simulink model "radia_streamfunction_optimization"  (R2026a)
settings: Solver=FixedStepDiscrete  StopTime=1  FixedStep=1
model workspace (MAT data in the model file):
  radia_streamfunction_adjoint_runner = radia.topopt.AdjointRunner
  radia_streamfunction_adjoint_runner.InitialDesign = [0.7; 0.7]
  radia_streamfunction_adjoint_runner.EvaluateFcn : function handle (value not decoded)
  radia_streamfunction_adjoint_runner.Options.LowerBounds = [0; 0]
  radia_streamfunction_adjoint_runner.Options.UpperBounds = [1; 1]
  radia_streamfunction_adjoint_runner.Options.MaxIterations = 40
  radia_streamfunction_adjoint_runner.Options.MoveLimit = [0.2; 0.2]
  radia_streamfunction_adjoint_runner.Metadata.domain = "stream-function"
  radia_streamfunction_adjoint_runner.Metadata.parameterization = "stream-function-coefficients"
  radia_streamfunction_adjoint_runner.Metadata.gradient = "analytic-adjoint"
  radia_streamfunction_adjoint_runner.Metadata.response_count = 2
  radia_streamfunction_adjoint_runner.Metadata.design_count = 2
  radia_streamfunction_adjoint_runner.Metadata.current_constraint_count = 1
settings Model: Creator=administrator  LastModifiedBy=administrator

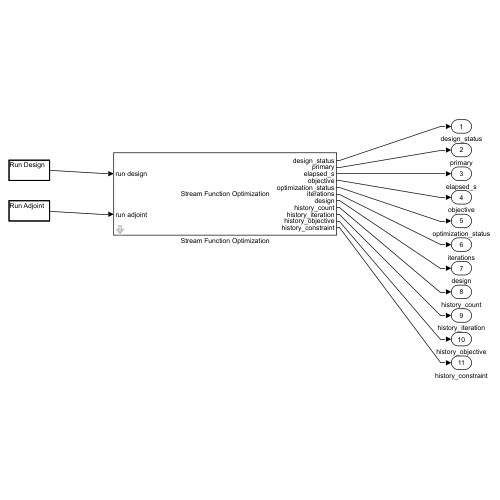
[thumbnail: Simulink's stored preview of the top-level diagram]
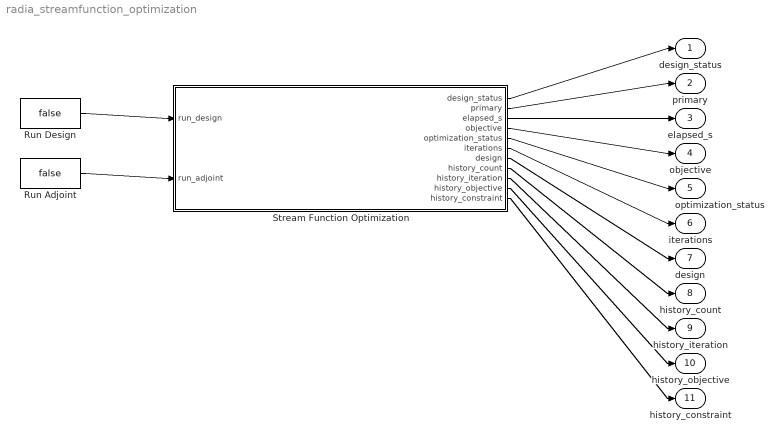
== system radia_streamfunction_optimization ==
  Run Adjoint : Constant  Value=false  OutDataTypeStr=boolean
  Run Design : Constant  Value=false  OutDataTypeStr=boolean
  Stream Function Optimization : Subsystem  mask{config_file='', run_root='C:\temp\radia_simulink', timeout_s=3600, python_executable='python', radia_streamfunction_adjoint_runner=radia_streamfunction_adjoint_runner, solver=mma, sample_time_s=1, history_capacity=64}
      mask prompts: config_file "Design configuration JSON"; run_root "Run artifact root"; timeout_s "Timeout (s)"; python_executable "Python executable"; radia_streamfunction_adjoint_runner "Stream-function adjoint runner"; solver "Optimizer"; sample_time_s "Sample time (s)"; history_capacity "History capacity"
      mask help: Stream-function design/Pareto batch plus analytic MMA/SQP coefficient optimization and Simulink-native history plots.
      mask init:
      | radia.simulink.configureStreamFunctionOptimizationSubsystem(gcb);
      mask TypeOptions solver: mma | sqp
      mask Display: disp('Stream Function Optimization');port_label('input',1,'run design');port_label('input',2,'run adjoint');port_label('output',1,'design_status');port_label('output',2,'primary');port_label('output',3,'elapsed_s');port_label('output',4,'objective');port_label('output',5,'optimization_status');port_label('output',6,'iterations');port_label('output',7,'design');port_label('output',8,'history_count');port_label('output',9,'history_iteration');port_label('output',10,'history_objective');port_label('output',11,'history_constraint');
  design_status : Outport
  primary : Outport  Port=2
  elapsed_s : Outport  Port=3
  objective : Outport  Port=4
  optimization_status : Outport  Port=5
  iterations : Outport  Port=6
  design : Outport  Port=7
  history_count : Outport  Port=8
  history_iteration : Outport  Port=9
  history_objective : Outport  Port=10
  history_constraint : Outport  Port=11
  wires:
  Run Design/1 -> Stream Function Optimization/1(run_design)
  Run Adjoint/1 -> Stream Function Optimization/2(run_adjoint)
  Stream Function Optimization/1(design_status) -> design_status/1
  Stream Function Optimization/2(primary) -> primary/1
  Stream Function Optimization/3(elapsed_s) -> elapsed_s/1
  Stream Function Optimization/4(objective) -> objective/1
  Stream Function Optimization/5(optimization_status) -> optimization_status/1
  Stream Function Optimization/6(iterations) -> iterations/1
  Stream Function Optimization/7(design) -> design/1
  Stream Function Optimization/8(history_count) -> history_count/1
  Stream Function Optimization/9(history_iteration) -> history_iteration/1
  Stream Function Optimization/10(history_objective) -> history_objective/1
  Stream Function Optimization/11(history_constraint) -> history_constraint/1

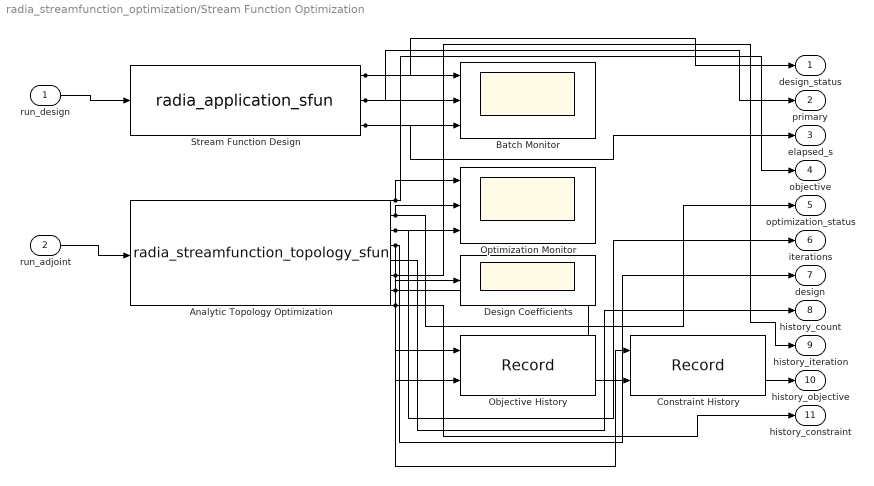
== system radia_streamfunction_optimization/Stream Function Optimization ==
  run_design : Inport  OutDataTypeStr=boolean
  run_adjoint : Inport  Port=2  OutDataTypeStr=boolean
  Analytic Topology Optimization : M-S-Function  FunctionName=radia_streamfunction_topology_sfun  Parameters=radia_streamfunction_adjoint_runner,1,64
  Batch Monitor : Scope  NumInputPorts=3
  Constraint History : Record  NumPorts=2.0  FileSettingsInternal="{\"entries\":[{\"content\":{\"excelSettings\":{\"content\":{},\"type\":\"Streamout.ExcelSettings\"},\"parquetSettings\":{\"content\":{},\"type\":\"Streamout.ParquetSettings\"}},\"type\":\"Streamout.FileSettingStorage\",\"uuid\":\"\"}],\"packageUris\":[\"http:\\/\\/schema.mathworks.com\\/mf0\\/streamout_blocks\\/R2020a\"],\"version\":\"1.0\"}"  FrameSettings=[0, 0]  Layout=[1 1]  SignalsInternal="{\"entries\":[{\"content\":{\"signals\":[{\"content\":{\"blockPath\":[],\"dimensions\":[1],\"domain\":\"\",\"lineColor\":\"#a2142f\",\"plots\":[ 1 ],\"port\":1,\"signalID\":1,\"signalName\":\"XY Graph:1\"},\"type\":\"RecordBlkView.Signal\",\"uuid\":\"\"},{\"content\":{\"blockPath\":[],\"dimensions\":[1],\"domain\":\"\",\"lineColor\":\"#139fff\",\"plots\":[ 1 ],\"port\":2,\"signalID\":2,\"signalName\":\"XY Graph:2\"},\"type\":\"RecordBlkView.Signal\",\"uuid\":\"\"}]},\"type\":\"RecordBlkView.InputSignals\",\"uuid\":\"\"}],\"packageUris\":[\"http:\\/\\/schema.mathworks.com\\/mf0\\/streamout_blocks\\/R2020a\"],\"version\":\"1.0\"}"  VisualizationBindings="{\"xyplotplugin\":{\"info\":[{\"series\":[{\"bindingParametersList\":[{\"parameter\":\"X-Axis\",\"signalID\":1,\"signalName\":\"XY Graph:1\"},{\"parameter\":\"Y-Axis\",\"signalID\":2,\"signalName\":\"XY Graph:2\"}],\"seriesID\":0}],\"subplotID\":1}]}}"  CompatibilityTag=XY
  Design Coefficients : Scope
  Objective History : Record  NumPorts=2.0  FileSettingsInternal="{\"entries\":[{\"content\":{\"excelSettings\":{\"content\":{},\"type\":\"Streamout.ExcelSettings\"},\"parquetSettings\":{\"content\":{},\"type\":\"Streamout.ParquetSettings\"}},\"type\":\"Streamout.FileSettingStorage\",\"uuid\":\"\"}],\"packageUris\":[\"http:\\/\\/schema.mathworks.com\\/mf0\\/streamout_blocks\\/R2020a\"],\"version\":\"1.0\"}"  FrameSettings=[0, 0]  Layout=[1 1]  SignalsInternal="{\"entries\":[{\"content\":{\"signals\":[{\"content\":{\"blockPath\":[],\"dimensions\":[1],\"domain\":\"\",\"lineColor\":\"#a2142f\",\"plots\":[ 1 ],\"port\":1,\"signalID\":1,\"signalName\":\"XY Graph:1\"},\"type\":\"RecordBlkView.Signal\",\"uuid\":\"\"},{\"content\":{\"blockPath\":[],\"dimensions\":[1],\"domain\":\"\",\"lineColor\":\"#139fff\",\"plots\":[ 1 ],\"port\":2,\"signalID\":2,\"signalName\":\"XY Graph:2\"},\"type\":\"RecordBlkView.Signal\",\"uuid\":\"\"}]},\"type\":\"RecordBlkView.InputSignals\",\"uuid\":\"\"}],\"packageUris\":[\"http:\\/\\/schema.mathworks.com\\/mf0\\/streamout_blocks\\/R2020a\"],\"version\":\"1.0\"}"  VisualizationBindings="{\"xyplotplugin\":{\"info\":[{\"series\":[{\"bindingParametersList\":[{\"parameter\":\"X-Axis\",\"signalID\":1,\"signalName\":\"XY Graph:1\"},{\"parameter\":\"Y-Axis\",\"signalID\":2,\"signalName\":\"XY Graph:2\"}],\"seriesID\":0}],\"subplotID\":1}]}}"  CompatibilityTag=XY
  Optimization Monitor : Scope  NumInputPorts=3
  Stream Function Design : M-S-Function  FunctionName=radia_application_sfun  Parameters='streamfunction','','C:\temp\radia_simulink',3600,'python'
  design_status : Outport
  primary : Outport  Port=2
  elapsed_s : Outport  Port=3
  objective : Outport  Port=4
  optimization_status : Outport  Port=5
  iterations : Outport  Port=6
  design : Outport  Port=7
  history_count : Outport  Port=8
  history_iteration : Outport  Port=9
  history_objective : Outport  Port=10
  history_constraint : Outport  Port=11
  wires:
  run_design/1 -> Stream Function Design/1
  run_adjoint/1 -> Analytic Topology Optimization/1
  Stream Function Design/1 -> design_status/1, Batch Monitor/1
  Stream Function Design/2 -> primary/1, Batch Monitor/2
  Stream Function Design/3 -> elapsed_s/1, Batch Monitor/3
  Analytic Topology Optimization/1 -> objective/1, Optimization Monitor/1
  Analytic Topology Optimization/2 -> optimization_status/1, Optimization Monitor/2
  Analytic Topology Optimization/3 -> iterations/1, Optimization Monitor/3
  Analytic Topology Optimization/4 -> design/1, Design Coefficients/1
  Analytic Topology Optimization/5 -> history_count/1
  Analytic Topology Optimization/6 -> history_iteration/1, Objective History/1, Constraint History/1
  Analytic Topology Optimization/7 -> history_objective/1, Objective History/2
  Analytic Topology Optimization/8 -> history_constraint/1, Constraint History/2
